simulink model "SILS_20170421"  (Simulink 10.2)
settings: Solver=ode4  StartTime=0.0  StopTime=20000  FixedStep=sim_dt  RelTol=1e-3  EnableMultiTasking=on
PreLoadFcn:
  | start
  | make_SILS
  | param_SW
  | param_sys
  | param_component
  | param_env
  | param_alignment
  | OEread
  | initialCondition
undefined symbols (not defined in the file or in its folder): ADSW, AOBC_dt, area, GAS_b2c, GGSW, GPperturbationSW, GYRO_b2c, MTQ_c2b, noise_sampling_rate, NSAS1_b2c, NSAS2_b2c, NSAS3_b2c, NSAS4_b2c, NSAS5_b2c, NSAS6_b2c, rem_mag, rem_magSW, RW_J, SRPSW, STT1_b2c_quat, STT_seed1, STT_x_noise, STT_y_noise, STT_z_noise
libraries: lib_util x23, lib_component x14, lib_env x9, aerolibutil x4, lib_orbittrance x3, aerolibtransform2 x1, sharedtransform x1
CloseFcn:
  | clean
settings Model: Creator=yamaurashusaku  LastModifiedBy=hapham
settings DataIOCC: LimitDataPoints=on  SaveFinalState=on  SaveFormat=StructureWithTime  SaveState=on  StateSaveName=tmp_raccel_xout
settings OptimizationCC: ExpressionDepthLimit=2147483647  EfficientMapNaN2IntZero=off  LifeSpan=auto
settings DebuggingCC: SolverPrmCheckMsg=warning  MultiTaskCondExecSysMsg=warning  RootOutportRequireBusObject=error  StateNameClashWarn=warning  StrictBusMsg=ErrorOnBusTreatedAsVector
settings HardwareCC: ProdBitPerPointer=64  ProdBitPerSizeT=64  ProdBitPerPtrDiffT=64  ProdLargestAtomicFloat=Float  ProdIntDivRoundTo=Zero  ProdEndianess=LittleEndian  ProdWordSize=64  ProdHWDeviceType=Intel->x86-64 (Windows64)  TargetBitPerPointer=64  TargetBitPerSizeT=64  TargetBitPerPtrDiffT=64  TargetLongLongMode=on  TargetIntDivRoundTo=Zero  TargetEndianess=LittleEndian  TargetWordSize=64  TargetHWDeviceType=MATLAB Host  ProdEqTarget=off
settings SFSimCC: SimUserSources=|
  | sfunc_nrlmsise00_wrapper.c
  | nrlmsise-00.c
  | nrlmsise-00_data.c
  | createHandle.c
  | globals.c
  | AOCS_Process.c
settings RTWCC: Description=Create Visual C/C++ Solution File for Simulink Coder  GenerateMakefile=off  TemplateMakefile=RTW.MSVCBuild  RTWVerbose=off  RTWUseSimCustomCode=on
settings RTWCC: CustomSource=|
  | sfunc_nrlmsise00_wrapper.c
  | nrlmsise-00.c
  | nrlmsise-00_data.c
  | createHandle.c
  | globals.c
  | AOCS_Process.c
settings CodeAppCC: GenerateComments=off  MaxIdLength=128  SimulinkBlockComments=off  StateflowObjectComments=off
settings GRTTargetCC: CombineOutputUpdateFcns=on  GRTInterface=off
settings ConfigComp: CovSFcnEnable=off

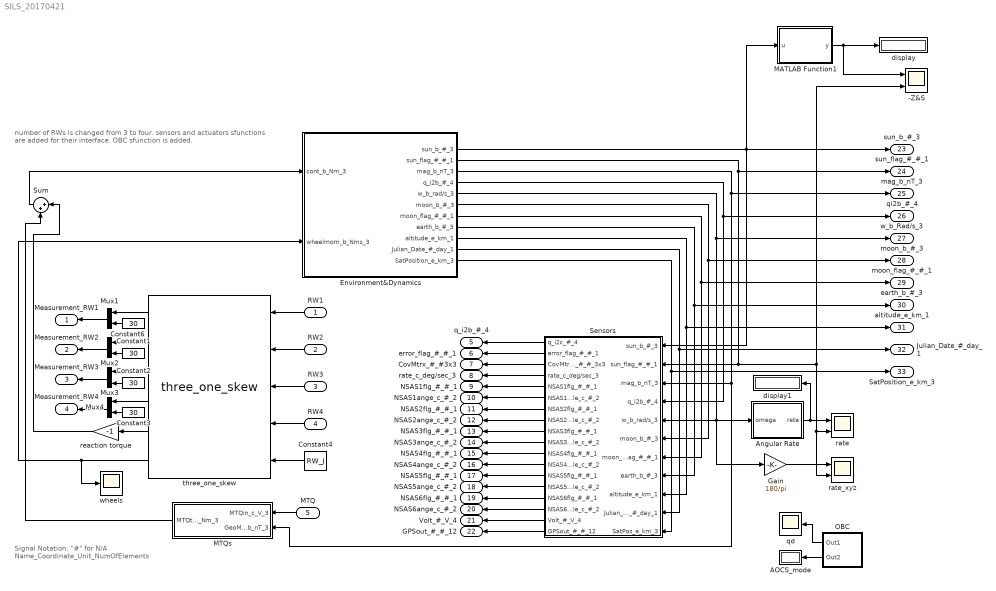
== system SILS_20170421 ==
  note: Signal Notation: "#" for N/A
      | Name_Coordinate_Unit_NumOfElements
  note: number of RWs is changed from 3 to four.
      | sensors and actuators sfunctions are added for their interface.
      | OBC sfunction is added.
  RW1 : Inport
  RW2 : Inport  Port=2
  RW3 : Inport  Port=3
  RW4 : Inport  Port=4
  MTQ : Inport  Port=5
  -Z&S : Scope  NumInputPorts=2
  AOCS_mode : Display
  Angular Rate : MATLAB Function  TreatAsAtomicUnit=on
  Constant{1..3,6} (4 alike) : Constant  Value=30
  Constant4 : Constant  Value=RW_J
  Environment&Dynamics : Subsystem
  Gain : Gain  Gain=180/pi
  MATLAB Function1 : MATLAB Function  TreatAsAtomicUnit=on
  MTQs : Subsystem
  Mux{1..4} (4 alike) : Mux  Inputs=2
  OBC : Subsystem
  Sensors : Subsystem
  Sum : Sum  Inputs=|++
  display : Display
  display1 : Display
  qd : Scope
  rate : Scope  NumInputPorts=2
  rate_xyz : Scope  NumInputPorts=2
  reaction torque : Gain  Gain=-1
  three_one_skew : lib_component/three_one_skew  SystemSampleTime=-1  VariantActivationTime=update diagram  Latency=0  AutoFrameSizeCalculation=off
  wheels : Scope
  Measurement_RW1 : Outport
  Measurement_RW2 : Outport  Port=2
  Measurement_RW3 : Outport  Port=3
  Measurement_RW4 : Outport  Port=4
  q_i2b_#_4 : Outport  Port=5
  error_flag_#_#_1 : Outport  Port=6
  CovMtrx_#_#3x3 : Outport  Port=7
  rate_c_deg/sec_3 : Outport  Port=8
  NSAS1flg_#_#_1 : Outport  Port=9
  NSAS1ange_c_#_2 : Outport  Port=10
  NSAS2flg_#_#_1 : Outport  Port=11
  NSAS2ange_c_#_2 : Outport  Port=12
  NSAS3flg_#_#_1 : Outport  Port=13
  NSAS3ange_c_#_2 : Outport  Port=14
  NSAS4flg_#_#_1 : Outport  Port=15
  NSAS4ange_c_#_2 : Outport  Port=16
  NSAS5flg_#_#_1 : Outport  Port=17
  NSAS5ange_c_#_2 : Outport  Port=18
  NSAS6flg_#_#_1 : Outport  Port=19
  NSAS6ange_c_#_2 : Outport  Port=20
  Volt_#_V_4 : Outport  Port=21
  GPSout_#_#_12 : Outport  Port=22
  sun_b_#_3 : Outport  Port=23
  sun_flag_#_#_1 : Outport  Port=24
  mag_b_nT_3 : Outport  Port=25
  qi2b_#_4 : Outport  Port=26
  w_b_Rad/s_3 : Outport  Port=27
  moon_b_#_3 : Outport  Port=28
  moon_flag_#_#_1 : Outport  Port=29
  earth_b_#_3 : Outport  Port=30
  altitude_e_km_1 : Outport  Port=31
  Julian_Date_#_day_1 : Outport  Port=32
  SatPosition_e_km_3 : Outport  Port=33
  wires:
  three_one_skew/6 -> Environment&Dynamics/2(wheelmom_b_Nms_3), wheels/1
  Environment&Dynamics/1(sun_b_#_3) -> sun_b_#_3/1, Sensors/1(sun_b_#_3), MATLAB Function1/1(u)
  Environment&Dynamics/2(sun_flag_#_#_1) -> sun_flag_#_#_1/1, -Z&S/2, rate/2, rate_xyz/2, Sensors/2(sun_flag_#_#_1)
  Environment&Dynamics/3(mag_b_nT_3) -> mag_b_nT_3/1, Sensors/3(mag_b_nT_3), MTQs/2(GeoMag_b_nT_3)
  Environment&Dynamics/4(q_i2b_#_4) -> qi2b_#_4/1, Sensors/4(q_i2b_#_4)
  Environment&Dynamics/5(w_b_rad/s_3) -> w_b_Rad/s_3/1, Angular Rate/1(omega), Sensors/5(w_b_rad/s_3), Gain/1
  Environment&Dynamics/6(moon_b_#_3) -> moon_b_#_3/1, Sensors/6(moon_b_#_3)
  Environment&Dynamics/7(moon_flag_#_#_1) -> moon_flag_#_#_1/1, Sensors/7(moon_flag_#_#_1)
  Environment&Dynamics/8(earth_b_#_3) -> earth_b_#_3/1, Sensors/8(earth_b_#_3)
  Environment&Dynamics/9(altitude_e_km_1) -> altitude_e_km_1/1, Sensors/9(altitude_e_km_1)
  Environment&Dynamics/10(Julian_Date_#_day_1) -> Julian_Date_#_day_1/1, Sensors/10(Julian_Date_#_day_1)
  Environment&Dynamics/11(SatPosition_e_km_3) -> SatPosition_e_km_3/1, Sensors/11(SatPos_e_km_3)
  three_one_skew/5 -> reaction torque/1
  MTQs/1(MTQtorque_b_Nm_3) -> Sum/2
  Sum/1 -> Environment&Dynamics/1(cont_b_Nm_3)
  OBC/1(Out1) -> qd/1
  MTQ/1 -> MTQs/1(MTQin_c_V_3)
  Mux1/1 -> Measurement_RW1/1
  three_one_skew/1 -> Mux1/1
  Constant6/1 -> Mux1/2
  Mux2/1 -> Measurement_RW2/1
  three_one_skew/2 -> Mux2/1
  Constant1/1 -> Mux2/2
  Mux3/1 -> Measurement_RW3/1
  three_one_skew/3 -> Mux3/1
  Constant2/1 -> Mux3/2
  Mux4/1 -> Measurement_RW4/1
  three_one_skew/4 -> Mux4/1
  Constant3/1 -> Mux4/2
  Constant4/1 -> three_one_skew/5
  reaction torque/1 -> Sum/1
  Gain/1 -> rate_xyz/1
  OBC/2(Out2) -> AOCS_mode/1
  Sensors/1(q_i2c_#_4) -> q_i2b_#_4/1
  Sensors/2(error_flag_#_#_1) -> error_flag_#_#_1/1
  Sensors/3(CovMtrx_#_#_3x3) -> CovMtrx_#_#3x3/1
  Sensors/4(rate_c_deg/sec_3) -> rate_c_deg/sec_3/1
  Sensors/5(NSAS1flg_#_#_1) -> NSAS1flg_#_#_1/1
  Sensors/6(NSAS1angle_c_#_2) -> NSAS1ange_c_#_2/1
  Sensors/8(NSAS2angle_c_#_2) -> NSAS2ange_c_#_2/1
  Sensors/9(NSAS3flg_#_#_1) -> NSAS3flg_#_#_1/1
  Sensors/10(NSAS3angle_c_#_2) -> NSAS3ange_c_#_2/1
  Sensors/11(NSAS4flg_#_#_1) -> NSAS4flg_#_#_1/1
  Sensors/12(NSAS4angle_c_#_2) -> NSAS4ange_c_#_2/1
  Angular Rate/1(rate) -> display1/1, rate/1
  MATLAB Function1/1(y) -> -Z&S/1, display/1
  RW1/1 -> three_one_skew/1
  RW2/1 -> three_one_skew/2
  RW3/1 -> three_one_skew/3
  RW4/1 -> three_one_skew/4
  Sensors/7(NSAS2flg_#_#_1) -> NSAS2flg_#_#_1/1
  Sensors/13(NSAS5flg_#_#_1) -> NSAS5flg_#_#_1/1
  Sensors/14(NSAS5angle_c_#_2) -> NSAS5ange_c_#_2/1
  Sensors/15(NSAS6flg_#_#_1) -> NSAS6flg_#_#_1/1
  Sensors/16(NSAS6angle_c_#_2) -> NSAS6ange_c_#_2/1
  Sensors/17(Volt_#_V_4) -> Volt_#_V_4/1
  Sensors/18(GPSout_#_#_12) -> GPSout_#_#_12/1

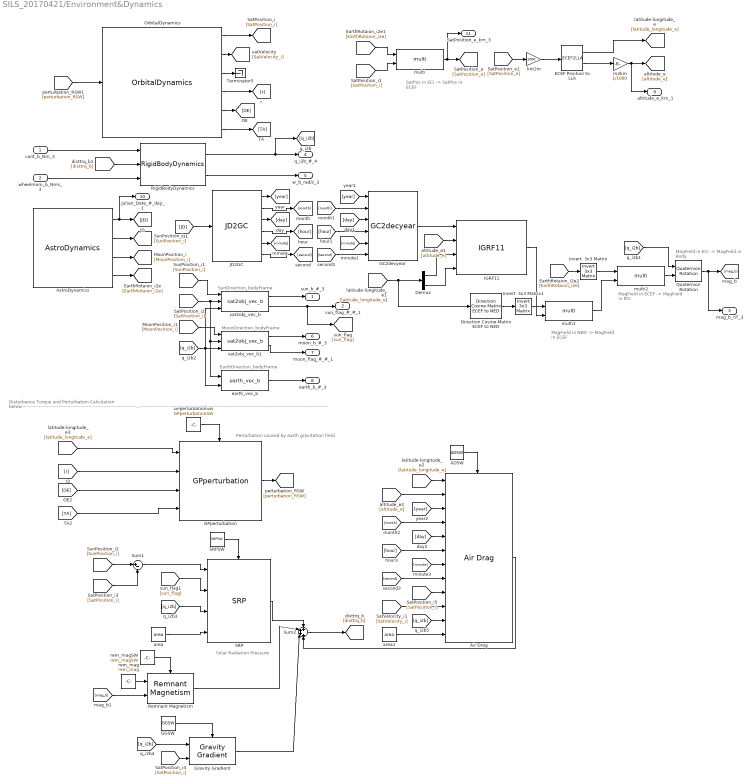
== system SILS_20170421/Environment&Dynamics ==
  note: MagField in ECI ->
      | MagField in Body
  note: MagField in ECEF ->
      | MagField in ECI
  note: MagField in NED ->
      | MagField in ECEF
  note: SatPos in ECI ->
      | SatPos in ECEF
  note: EarthDirection_bodyFrame
  note: MoonDirection_bodyFrame
  note: SunDirection_bodyFrame
  note: Disturbance Torque and Perturbation Calculation below-------------------------------------------------------------------------------------------------------------------------------------------------------------------------------------------------------------------------------------------------------------------------------------------------------------------------------------------------------
  note: Perturbation caused by earth gravitation field
  note: Solar Radiation Pressure
  cont_b_Nm_3 : Inport
  wheelmom_b_Nms_3 : Inport  Port=2
  ADSW : Constant  Value=ADSW
  Air Drag : lib_env/Environment&Dynamics/Air Drag  SystemSampleTime=-1  VariantActivationTime=update diagram  Latency=0  AutoFrameSizeCalculation=off
  AstroDynamics : lib_env/Environment&Dynamics/AstroDynamics  SystemSampleTime=-1  VariantActivationTime=update diagram  Latency=0  AutoFrameSizeCalculation=off
  Demux : Demux  Outputs=2
  Direction Cosine Matrix ECEF to NED : aerolibtransform2/Direction Cosine Matrix ECEF to NED
      settings: SourceProductBaseCode=AE
  ECEF Position to LLA : ECEF2LLA  R=6378137
  GC2decyear : lib_util/GC2decyear  SystemSampleTime=-1  VariantActivationTime=update diagram  Latency=0  AutoFrameSizeCalculation=off
  GGSW : Constant  Value=GGSW
  GPperturbation : lib_env/Environment&Dynamics/GPperturbation  SystemSampleTime=-1  VariantActivationTime=update diagram  Latency=0  AutoFrameSizeCalculation=off
  GPperturbationSW : Constant  Value=GPperturbationSW
  Gravity Gradient : lib_env/Environment&Dynamics/Gravity Gradient  SystemSampleTime=-1  VariantActivationTime=update diagram  Latency=0  AutoFrameSizeCalculation=off
  IGRF11 : lib_env/IGRF11  SystemSampleTime=-1  VariantActivationTime=update diagram  Latency=0  AutoFrameSizeCalculation=off
  Invert  3x3 Matrix : aerolibutil/Invert  3x3 Matrix
  Invert  3x3 Matrix1 : aerolibutil/Invert  3x3 Matrix
  JD2GC : lib_util/JD2GC  SystemSampleTime=-1  VariantActivationTime=update diagram  Latency=0  AutoFrameSizeCalculation=off
  OrbitalDynamics : lib_env/Environment&Dynamics/OrbitalDynamics  SystemSampleTime=-1  VariantActivationTime=update diagram  Latency=0  AutoFrameSizeCalculation=off
  Quaternion Rotation : aerolibutil/Quaternion Rotation
  Remnant Magnetism : lib_env/Environment&Dynamics/Remnant Magnetism  SystemSampleTime=-1  VariantActivationTime=update diagram  Latency=0  AutoFrameSizeCalculation=off
  RigidBodyDynamics : lib_env/Environment&Dynamics/RigidBodyDynamics  SystemSampleTime=-1  VariantActivationTime=update diagram  Latency=0  AutoFrameSizeCalculation=off
  SRP : lib_env/Environment&Dynamics/SRP  SystemSampleTime=-1  VariantActivationTime=update diagram  Latency=0  AutoFrameSizeCalculation=off
  SRPSW : Constant  Value=SRPSW
  Sum1 : Sum  Inputs=|+-
  Sum2 : Sum  Inputs=++++
  Terminator5 : Terminator
  area : Constant  Value=area
  area1 : Constant  Value=area
  earth_vec_b : lib_orbittrance/earth_vec_b  SystemSampleTime=-1  VariantActivationTime=update diagram  Latency=0  AutoFrameSizeCalculation=off
  km2m : Gain  Gain=1000
  m2km : Gain  Gain=1/1000
  multi : lib_util/multi  SystemSampleTime=-1  VariantActivationTime=update diagram  Latency=0  AutoFrameSizeCalculation=off
  multi1 : lib_util/multi  SystemSampleTime=-1  VariantActivationTime=update diagram  Latency=0  AutoFrameSizeCalculation=off
  multi2 : lib_util/multi  SystemSampleTime=-1  VariantActivationTime=update diagram  Latency=0  AutoFrameSizeCalculation=off
  rem_mag : Constant  Value=rem_mag
  rem_magSW : Constant  Value=rem_magSW
  sat2obj_vec_b : lib_orbittrance/sat2obj_vec_b  SystemSampleTime=-1  VariantActivationTime=update diagram  Latency=0  AutoFrameSizeCalculation=off
  sat2obj_vec_b1 : lib_orbittrance/sat2obj_vec_b  SystemSampleTime=-1  VariantActivationTime=update diagram  Latency=0  AutoFrameSizeCalculation=off
  sun_b_#_3 : Outport
  sun_flag_#_#_1 : Outport  Port=2
  mag_b_nT_3 : Outport  Port=3
  q_i2b_#_4 : Outport  Port=4
  w_b_rad/s_3 : Outport  Port=5
  moon_b_#_3 : Outport  Port=6
  moon_flag_#_#_1 : Outport  Port=7
  earth_b_#_3 : Outport  Port=8
  altitude_e_km_1 : Outport  Port=9
  Julian_Date_#_day_1 : Outport  Port=10
  SatPosition_e_km_3 : Outport  Port=11
  wires:
  RigidBodyDynamics/1 -> q_i2b_#_4/1, [q_i2b]
  RigidBodyDynamics/2 -> w_b_rad/s_3/1
  cont_b_Nm_3/1 -> RigidBodyDynamics/1
  wheelmom_b_Nms_3/1 -> RigidBodyDynamics/3
  AstroDynamics/1 -> [JD], Julian_Date_#_day_1/1
  AstroDynamics/4 -> [EarthRotaion_i2e]
  [second] -> GC2decyear/6
  [minute] -> GC2decyear/5
  [hour] -> GC2decyear/4
  [day] -> GC2decyear/3
  [month] -> GC2decyear/2
  [year] -> GC2decyear/1
  JD2GC/6 -> [second]
  JD2GC/5 -> [minute]
  JD2GC/4 -> [hour]
  JD2GC/3 -> [day]
  JD2GC/2 -> [month]
  JD2GC/1 -> [year]
  Quaternion Rotation/1 -> mag_b_nT_3/1, [mag_b]
  [q_i2b] -> Quaternion Rotation/1
  multi2/1 -> Quaternion Rotation/2
  multi1/1 -> multi2/2
  Invert  3x3 Matrix/1 -> multi2/1
  [EarthRotaion_i2e] -> Invert  3x3 Matrix/1
  IGRF11/1 -> multi1/2
  Invert  3x3 Matrix1/1 -> multi1/1
  Direction Cosine Matrix ECEF to NED/1 -> Invert  3x3 Matrix1/1
  Demux/2 -> IGRF11/4
  Demux/1 -> IGRF11/3
  [altitude_e] -> IGRF11/2
  [latitude_longitude_e] -> Direction Cosine Matrix ECEF to NED/1, Demux/1
  [JD] -> JD2GC/1
  GC2decyear/1 -> IGRF11/1
  ECEF Position to LLA/1 -> [latitude_longitude_e]
  m2km/1 -> [altitude_e], altitude_e_km_1/1
  ECEF Position to LLA/2 -> m2km/1
  km2m/1 -> ECEF Position to LLA/1
  [SatPosition_e] -> km2m/1
  multi/1 -> [SatPosition_e], SatPosition_e_km_3/1
  [SatPosition_i] -> multi/2
  [EarthRotaion_i2e] -> multi/1
  OrbitalDynamics/1 -> [SatPosition_i]
  OrbitalDynamics/2 -> [SatVelocity_i]
  OrbitalDynamics/4 -> [r]
  OrbitalDynamics/5 -> [OE]
  OrbitalDynamics/6 -> [TA]
  AstroDynamics/2 -> [SunPosition_i]
  AstroDynamics/3 -> [MoonPosition_i]
  earth_vec_b/1 -> earth_b_#_3/1
  sat2obj_vec_b1/2 -> moon_flag_#_#_1/1
  sat2obj_vec_b1/1 -> moon_b_#_3/1
  sat2obj_vec_b/1 -> sun_b_#_3/1
  sat2obj_vec_b/2 -> sun_flag_#_#_1/1, [sun_flag]
  [SunPosition_i] -> sat2obj_vec_b/1
  [MoonPosition_i] -> sat2obj_vec_b1/1
  [q_i2b] -> sat2obj_vec_b/3, earth_vec_b/2, sat2obj_vec_b1/3
  [SatPosition_i] -> sat2obj_vec_b/2, sat2obj_vec_b1/2, earth_vec_b/1
  OrbitalDynamics/3 -> Terminator5/1
  GPperturbation/1 -> [perturbation_RSW]
  Gravity Gradient/1 -> Sum2/3
  Remnant Magnetism/1 -> Sum2/2
  [latitude_longitude_e] -> GPperturbation/1
  [r] -> GPperturbation/2
  [OE] -> GPperturbation/3
  [TA] -> GPperturbation/4
  GPperturbationSW/1 -> GPperturbation/Enable
  Sum1/1 -> SRP/1
  [sun_flag] -> SRP/2
  area/1 -> SRP/4
  [q_i2b] -> SRP/3
  [SatPosition_i] -> Sum1/2
  [SunPosition_i] -> Sum1/1
  SRPSW/1 -> SRP/Enable
  rem_mag/1 -> Remnant Magnetism/1
  [mag_b] -> Remnant Magnetism/2
  rem_magSW/1 -> Remnant Magnetism/Enable
  Sum2/1 -> [disttrq_b]
  SRP/1 -> Sum2/1
  [q_i2b] -> Gravity Gradient/1
  [SatPosition_i] -> Gravity Gradient/2
  GGSW/1 -> Gravity Gradient/Enable
  [latitude_longitude_e] -> Air Drag/1
  [altitude_e] -> Air Drag/2
  [month] -> Air Drag/4
  [day] -> Air Drag/5
  [hour] -> Air Drag/6
  [minute] -> Air Drag/7
  [second] -> Air Drag/8
  [SatPosition_i] -> Air Drag/9
  [SatVelocity_i] -> Air Drag/10
  area1/1 -> Air Drag/12
  [q_i2b] -> Air Drag/11
  [year] -> Air Drag/3
  ADSW/1 -> Air Drag/Enable
  Air Drag/1 -> Sum2/4
  [disttrq_b] -> RigidBodyDynamics/2
  [perturbation_RSW] -> OrbitalDynamics/1

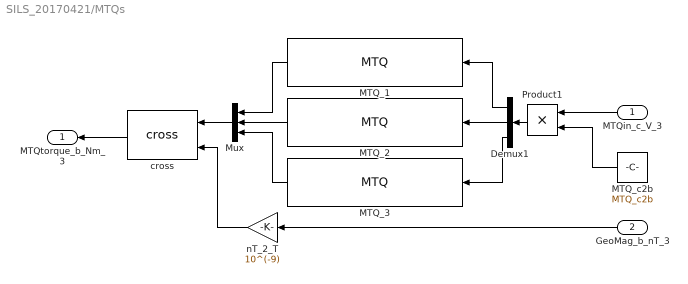
== system SILS_20170421/MTQs ==
  MTQin_c_V_3 : Inport
  GeoMag_b_nT_3 : Inport  Port=2
  Demux1 : Demux  Outputs=3
  MTQ_1 : lib_component/MTQ  SystemSampleTime=-1  VariantActivationTime=update diagram  Latency=0  AutoFrameSizeCalculation=off
  MTQ_2 : lib_component/MTQ  SystemSampleTime=-1  VariantActivationTime=update diagram  Latency=0  AutoFrameSizeCalculation=off
  MTQ_3 : lib_component/MTQ  SystemSampleTime=-1  VariantActivationTime=update diagram  Latency=0  AutoFrameSizeCalculation=off
  MTQ_c2b : Constant  Value=MTQ_c2b
  Mux : Mux  Inputs=3
  Product1 : Product  RndMeth=Zero
  cross : lib_util/cross  SystemSampleTime=-1  VariantActivationTime=update diagram  Latency=0  AutoFrameSizeCalculation=off
  nT_2_T : Gain  Gain=10^(-9)
  MTQtorque_b_Nm_3 : Outport
  wires:
  MTQ_1/1 -> Mux/1
  MTQ_2/1 -> Mux/2
  MTQ_3/1 -> Mux/3
  Mux/1 -> cross/1
  Demux1/1 -> MTQ_1/1
  Demux1/2 -> MTQ_2/1
  Demux1/3 -> MTQ_3/1
  nT_2_T/1 -> cross/2
  GeoMag_b_nT_3/1 -> nT_2_T/1
  MTQ_c2b/1 -> Product1/2
  Product1/1 -> Demux1/1
  MTQin_c_V_3/1 -> Product1/1
  cross/1 -> MTQtorque_b_Nm_3/1

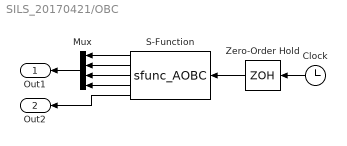
== system SILS_20170421/OBC ==
  Clock : Clock
  Mux : Mux
  S-Function : S-Function  FunctionName=sfunc_AOBC  SFunctionDeploymentMode=off  EnableBusSupport=off
  Zero-Order Hold : ZeroOrderHold  SampleTime=AOBC_dt
  Out1 : Outport
  Out2 : Outport  Port=2
  wires:
  Clock/1 -> Zero-Order Hold/1
  Zero-Order Hold/1 -> S-Function/1
  S-Function/1 -> Mux/1
  S-Function/2 -> Mux/2
  S-Function/3 -> Mux/3
  S-Function/4 -> Mux/4
  Mux/1 -> Out1/1
  S-Function/5 -> Out2/1

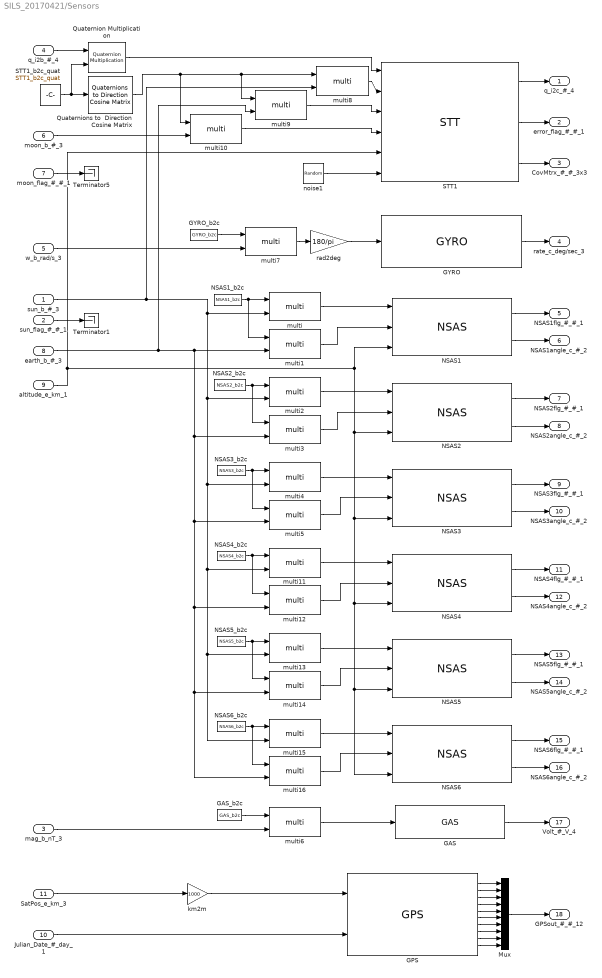
== system SILS_20170421/Sensors ==
  sun_b_#_3 : Inport
  sun_flag_#_#_1 : Inport  Port=2
  mag_b_nT_3 : Inport  Port=3
  q_i2b_#_4 : Inport  Port=4
  w_b_rad/s_3 : Inport  Port=5
  moon_b_#_3 : Inport  Port=6
  moon_flag_#_#_1 : Inport  Port=7
  earth_b_#_3 : Inport  Port=8
  altitude_e_km_1 : Inport  Port=9
  Julian_Date_#_day_1 : Inport  Port=10
  SatPos_e_km_3 : Inport  Port=11
  GAS : lib_component/GAS  SystemSampleTime=-1  VariantActivationTime=update diagram  Latency=0  AutoFrameSizeCalculation=off
  GAS_b2c : Constant  Value=GAS_b2c  VectorParams1D=off
  GPS : lib_component/GPS  SystemSampleTime=-1  VariantActivationTime=update diagram  Latency=0  AutoFrameSizeCalculation=off
  GYRO : lib_component/GYRO  SystemSampleTime=-1  VariantActivationTime=update diagram  Latency=0  AutoFrameSizeCalculation=off
  GYRO_b2c : Constant  Value=GYRO_b2c  VectorParams1D=off
  Mux : Mux  Inputs=10
  NSAS{1..6} (6 alike) : lib_component/NSAS  SystemSampleTime=-1  VariantActivationTime=update diagram  Latency=0  AutoFrameSizeCalculation=off
  NSAS1_b2c : Constant  Value=NSAS1_b2c  VectorParams1D=off
  NSAS2_b2c : Constant  Value=NSAS2_b2c  VectorParams1D=off
  NSAS3_b2c : Constant  Value=NSAS3_b2c  VectorParams1D=off
  NSAS4_b2c : Constant  Value=NSAS4_b2c  VectorParams1D=off
  NSAS5_b2c : Constant  Value=NSAS5_b2c  VectorParams1D=off
  NSAS6_b2c : Constant  Value=NSAS6_b2c  VectorParams1D=off
  Quaternion Multiplication : aerolibutil/Quaternion Multiplication
  Quaternions to  Direction Cosine Matrix : sharedtransform/Quaternions to  Direction Cosine Matrix  aMode=aMode
      settings: SourceProductBaseCode=AE,PW,MT,UV,VE,VP
  STT1 : lib_component/STT  SystemSampleTime=-1  VariantActivationTime=update diagram  Latency=0  AutoFrameSizeCalculation=off
  STT1_b2c_quat : Constant  Value=STT1_b2c_quat
  Terminator1 : Terminator
  Terminator5 : Terminator
  km2m : Gain  Gain=1000
  multi{,1..16} (17 alike) : lib_util/multi  SystemSampleTime=-1  VariantActivationTime=update diagram  Latency=0  AutoFrameSizeCalculation=off
  noise1 : RandomNumber  Mean=[0 0 0]  Variance=[STT_x_noise*STT_x_noise STT_y_noise*STT_y_noise STT_z_noise*STT_z_noise]  Seed=STT_seed1  SampleTime=noise_sampling_rate
  rad2deg : Gain  Gain=180/pi
  q_i2c_#_4 : Outport
  error_flag_#_#_1 : Outport  Port=2
  CovMtrx_#_#_3x3 : Outport  Port=3
  rate_c_deg/sec_3 : Outport  Port=4
  NSAS1flg_#_#_1 : Outport  Port=5
  NSAS1angle_c_#_2 : Outport  Port=6
  NSAS2flg_#_#_1 : Outport  Port=7
  NSAS2angle_c_#_2 : Outport  Port=8
  NSAS3flg_#_#_1 : Outport  Port=9
  NSAS3angle_c_#_2 : Outport  Port=10
  NSAS4flg_#_#_1 : Outport  Port=11
  NSAS4angle_c_#_2 : Outport  Port=12
  NSAS5flg_#_#_1 : Outport  Port=13
  NSAS5angle_c_#_2 : Outport  Port=14
  NSAS6flg_#_#_1 : Outport  Port=15
  NSAS6angle_c_#_2 : Outport  Port=16
  Volt_#_V_4 : Outport  Port=17
  GPSout_#_#_12 : Outport  Port=18
  wires:
  Mux/1 -> GPSout_#_#_12/1
  GAS/1 -> Volt_#_V_4/1
  NSAS3/2 -> NSAS3angle_c_#_2/1
  NSAS3/1 -> NSAS3flg_#_#_1/1
  NSAS2/2 -> NSAS2angle_c_#_2/1
  NSAS2/1 -> NSAS2flg_#_#_1/1
  NSAS1/2 -> NSAS1angle_c_#_2/1
  NSAS1/1 -> NSAS1flg_#_#_1/1
  GYRO/1 -> rate_c_deg/sec_3/1
  STT1/3 -> CovMtrx_#_#_3x3/1
  STT1/2 -> error_flag_#_#_1/1
  STT1/1 -> q_i2c_#_4/1
  moon_b_#_3/1 -> multi10/2
  GYRO_b2c/1 -> multi7/1
  w_b_rad/s_3/1 -> multi7/2
  mag_b_nT_3/1 -> multi6/2
  GAS_b2c/1 -> multi6/1
  NSAS3_b2c/1 -> multi5/1, multi4/1
  multi5/1 -> NSAS3/2
  NSAS2_b2c/1 -> multi3/1, multi2/1
  NSAS1_b2c/1 -> multi1/1, multi/1
  multi1/1 -> NSAS1/2
  multi9/1 -> STT1/3
  GPS/10 -> Mux/10
  GPS/9 -> Mux/9
  GPS/8 -> Mux/8
  GPS/7 -> Mux/7
  GPS/6 -> Mux/6
  GPS/5 -> Mux/5
  GPS/4 -> Mux/4
  GPS/3 -> Mux/3
  GPS/2 -> Mux/2
  GPS/1 -> Mux/1
  SatPos_e_km_3/1 -> km2m/1
  Julian_Date_#_day_1/1 -> GPS/2
  multi10/1 -> STT1/4
  multi8/1 -> STT1/2
  multi4/1 -> NSAS3/1
  multi3/1 -> NSAS2/2
  multi2/1 -> NSAS2/1
  multi6/1 -> GAS/1
  multi/1 -> NSAS1/1
  rad2deg/1 -> GYRO/1
  multi7/1 -> rad2deg/1
  km2m/1 -> GPS/1
  q_i2b_#_4/1 -> Quaternion Multiplication/1
  Quaternion Multiplication/1 -> STT1/1
  STT1_b2c_quat/1 -> Quaternion Multiplication/2, Quaternions to  Direction Cosine Matrix/1
  Quaternions to  Direction Cosine Matrix/1 -> multi10/1, multi9/1, multi8/1
  noise1/1 -> STT1/6
  moon_flag_#_#_1/1 -> Terminator5/1
  sun_flag_#_#_1/1 -> Terminator1/1
  NSAS4_b2c/1 -> multi11/1, multi12/1
  multi12/1 -> NSAS4/2
  multi11/1 -> NSAS4/1
  NSAS4/1 -> NSAS4flg_#_#_1/1
  NSAS4/2 -> NSAS4angle_c_#_2/1
  NSAS5_b2c/1 -> multi14/1, multi13/1
  multi14/1 -> NSAS5/2
  multi13/1 -> NSAS5/1
  NSAS5/1 -> NSAS5flg_#_#_1/1
  NSAS5/2 -> NSAS5angle_c_#_2/1
  NSAS6_b2c/1 -> multi16/1, multi15/1
  multi16/1 -> NSAS6/2
  multi15/1 -> NSAS6/1
  altitude_e_km_1/1 -> NSAS6/3, NSAS5/3, NSAS4/3, NSAS3/3, NSAS2/3, NSAS1/3, STT1/5
  earth_b_#_3/1 -> multi5/2, multi14/2, multi16/2, multi12/2, multi3/2, multi1/2, multi9/2
  sun_b_#_3/1 -> multi4/2, multi11/2, multi13/2, multi15/2, multi2/2, multi/2, multi8/2
  NSAS6/1 -> NSAS6flg_#_#_1/1
  NSAS6/2 -> NSAS6angle_c_#_2/1

== matlab function Angular Rate ==
  data: omega input double; rate output double
function rate = fcn(omega)
%#codegen

rate = sqrt(omega(1)^2+omega(2)^2+omega(3)^2) *180/pi;

== matlab function MATLAB Function1 ==
  data: u input double; y output double
function y = fcn(u)
%#codegen

v = [0; 0; -1];

u = u / norm(u);
v = v / norm(v);

costheta = u' * v;
if costheta > 1
    costheta = 1;
end
if costheta < -1
    costheta = -1;
end

y = acos(costheta) / pi * 180;
